simulink model "p03"  (R2016a)
settings: Solver=VariableStepAuto  StartTime=0.0  StopTime=10.0  RelTol=1e-3
libraries: simulink x1
settings Model: Creator=YYJ-PC  LastModifiedBy=YYJ-PC

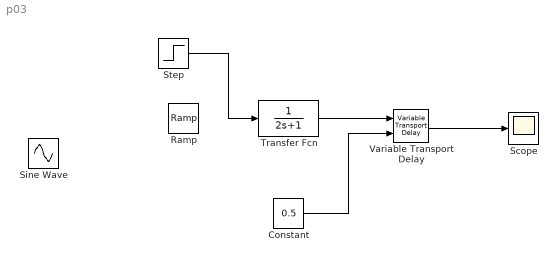
== system p03 ==
  Constant : Constant  Value=0.5
  Ramp : simulink/Sources/Ramp  slope=1  start=0  X0=0
  Scope : Scope
  Sine Wave : Sin  SampleTime=0
  Step : Step  Time=0  SampleTime=0
  Transfer Fcn : TransferFcn  Denominator=[2 1]
  Variable Transport Delay : VariableTransportDelay  MaximumDelay=10
  wires:
  Transfer Fcn/1 -> Variable Transport Delay/1
  Constant/1 -> Variable Transport Delay/2
  Variable Transport Delay/1 -> Scope/1
  Step/1 -> Transfer Fcn/1
